simulink model "bsm2_ol_test"  (R2023b)
settings: Solver=ode15s  StartTime=0.0  StopTime=50  FixedStep=0.01  RelTol=1e-5  AbsTol=1e-8
values from neighbouring files (symbols this model uses):
  ACTIVATE = [ 0 ]    [init_bsm1.m]    (also in init_bsm2.m)
  carb1 = 0    [reginit_bsm1.m]    (also in reginit_bsm2.m = 2)
  carb2 = 0    [reginit_bsm1.m]    (also in reginit_bsm2.m)
  carb3 = 0    [reginit_bsm1.m]    (also in reginit_bsm2.m)
  carb4 = 0    [reginit_bsm1.m]    (also in reginit_bsm2.m)
  carb5 = 0    [reginit_bsm1.m]    (also in reginit_bsm2.m)
  KLa1 = 0    [reginit_bsm1.m]    (also in reginit_bsm2.m)
  KLa2 = 0    [reginit_bsm1.m]    (also in reginit_bsm2.m)
  KLa3 = 240    [reginit_bsm1.m]    (also in reginit_bsm2.m = 120)
  KLa4 = 240    [reginit_bsm1.m]    (also in reginit_bsm2.m = 120)
  KLa5 = 84    [reginit_bsm1.m]    (also in reginit_bsm2.m = 60)
  PAR_P = [ f_corr  f_X  t_m  f_PS ]    [primclarinit_bsm2.m]
  Qbypass = 60000    [reginit_bsm1.m]    (also in reginit_bsm2.m)
  QbypassAS = 0    [reginit_bsm1.m]    (also in reginit_bsm2.m)
  Qbypassplant = 1    [reginit_bsm1.m]    (also in reginit_bsm2.m)
  Qstorage = 0    [reginit_bsm1.m]    (also in reginit_bsm2.m)
  Qstorage2AS = 0    [reginit_bsm1.m]    (also in reginit_bsm2.m)
  Qthickener2AS = 0    [reginit_bsm1.m]    (also in reginit_bsm2.m)
  T = 0.0001    [hyddelayinit_bsm2.m]
  TEMPMODEL = [ 0 ]    [init_bsm1.m]    (also in init_bsm2.m)
  VOL_P = 900    [primclarinit_bsm2.m]
  XINIT_P = [ S_I_P  S_S_P  X_I_P  X_S_P  X_BH_P  X_BA_P  X_P_P  S_O_P  S_NO_P  S_NH_P  S_ND_P  X_ND_P  S_ALK_P TSS_P Q_P T_P S_D1_P S_D2_P S_D3_P X_D4_P X_D5_P ]    [primclarinit_bsm2.m]
  XINITDELAY = [ S_I_ASin  S_S_ASin  X_I_ASin  X_S_ASin  X_BH_ASin  X_BA_ASin  X_P_ASin  S_O_ASin  S_NO_ASin  S_NH_ASin  S_ND_ASin  X_ND_ASin  S_ALK_ASin TSS_ASin Q_ASin T_ASin S_D1_ASin S_D2_ASin S_D3_ASin X_D4_ASin X_D5_ASin ]    [hyddelayinit_bsm2.m]
  XINITDELAYPRIMARY = [ S_I_Pin  S_S_Pin  X_I_Pin  X_S_Pin  X_BH_Pin  X_BA_Pin  X_P_Pin  S_O_Pin  S_NO_Pin  S_NH_Pin  S_ND_Pin  X_ND_Pin  S_ALK_Pin TSS_Pin Q_Pin T_Pin S_D1_Pin S_D2_Pin S_D3_Pin X_D4_Pin X_D5_Pin ]    [hyddelayinit_bsm2.m]
  XVEKTOR_P = [0  0  1  1  1  1  1  0  0  0  0  1  0  0  0  0  0  0  0  1  1]    [primclarinit_bsm2.m]
undefined symbols (not defined in the file or in its folder): DIM, LAYER, MODELTYPE, PAR1, PAR2, PAR3, PAR4, PAR5, Qintr, Qr, Qw, SETTLERINIT, SETTLERPAR, SOSAT1, SOSAT2, SOSAT3, SOSAT4, SOSAT5, TIMEDELAY_S, VOL1, VOL2, VOL3, VOL4, VOL5, VOL_INIT_S, VOL_S, XINIT1, XINIT2, XINIT3, XINIT4, XINIT5, XINITSTORAGE
settings Model: Creator=ielulf  LastModifiedBy=miederer
settings SolverCC: AutoScaleAbsTol=off  AlgebraicLoopSolver=TrustRegion
settings DataIOCC: InitialState=xFinal  SaveFormat=Array  SignalLoggingSaveFormat=ModelDataLogs  SaveOutput=off  ReturnWorkspaceOutputs=off  TimeSaveName=t  SignalLoggingName=sigsOut  OutputOption=SpecifiedOutputTimes  OutputTimes=[0:(1/96):50]
settings OptimizationCC: BlockReduction=off  BooleanDataType=off  OptimizeBlockIOStorage=off  BufferReuse=off  GlobalBufferReuse=off  ExpressionFolding=off  LocalBlockOutputs=off  InitFltsAndDblsToZero=on  LifeSpan=inf  OptimizeDataStoreBuffers=off  BusAssignmentInplaceUpdate=off
settings DebuggingCC: SaveWithParameterizedLinksMsg=none  UnderspecifiedInitializationDetection=Classic  MergeDetectMultiDrivingBlocksExec=none  SignalResolutionControl=TryResolveAllWithWarning  InheritedTsInSrcMsg=none  MultiTaskDSMMsg=warning  MultiTaskCondExecSysMsg=none  FcnCallInpInsideContextMsg=warning  UnconnectedInputMsg=warning  UnconnectedLineMsg=warning  SFUnexpectedBacktrackingDiag=warning  SFNoUnconditionalDefaultTransitionDiag=warning  SFExecutionAtInitializationDiag=none  ArithmeticOperatorsInVariantConditions=warning
settings HardwareCC: ProdBitPerPointer=32  ProdBitPerSizeT=32  ProdBitPerPtrDiffT=32  ProdLargestAtomicFloat=None  ProdIntDivRoundTo=Undefined  ProdEndianess=Unspecified  ProdWordSize=32  ProdHWDeviceType=32-bit Generic  TargetUnknown=on
settings ModelReferenceCC: EnableRefExpFcnMdlSchedulingChecks=on  PropagateSignalLabelsOutOfModel=off
settings RTWCC: TemplateMakefile=grt_unix.tmf
settings CodeAppCC: StateflowObjectComments=on
settings GRTTargetCC: TargetFcnLib=ansi_tfl_tmw.mat  TargetLangStandard=C89/C90 (ANSI)  CombineOutputUpdateFcns=off  GRTInterface=on
settings ConfigComp: CovMetricSettings=dw  CovSaveCumulativeToWorkspaceVar=on  CovSaveSingleToWorkspaceVar=on

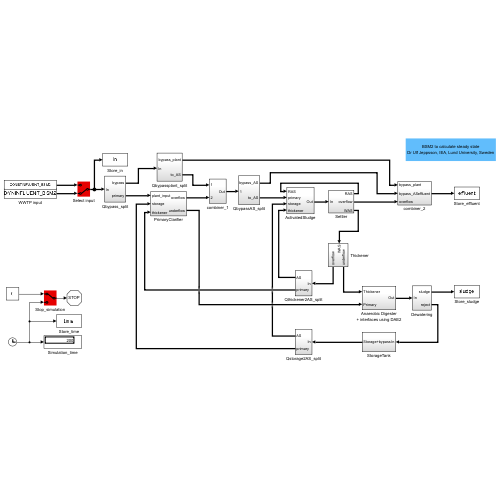
[thumbnail: Simulink's stored preview of the top-level diagram]
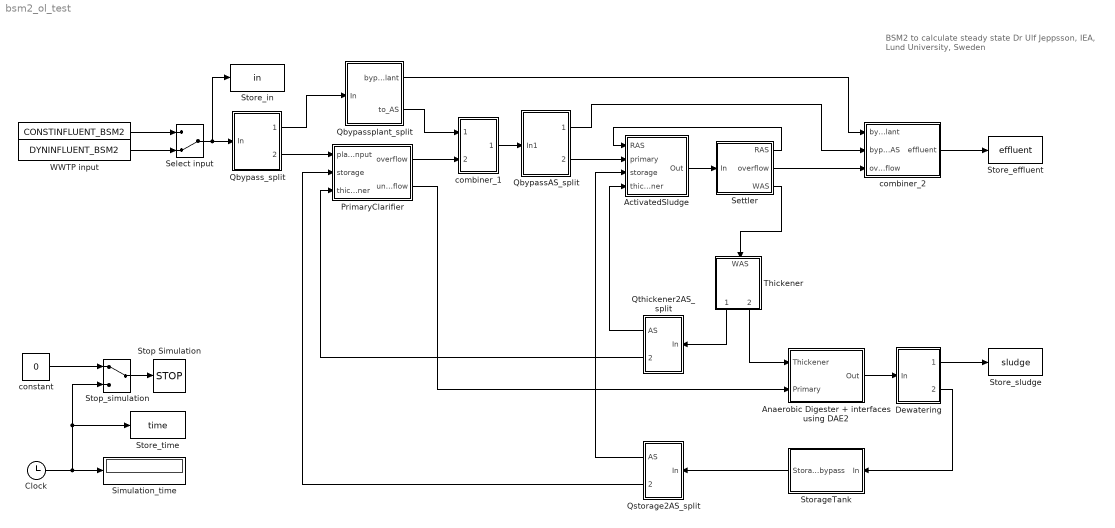
== system bsm2_ol_test ==
  note: BSM2 to calculate steady state
      |  Dr Ulf Jeppsson, IEA, Lund University, Sweden
  " " : FromWorkspace  VariableName=CONSTINFLUENT_BSM2  SampleTime=-1  ZeroCross=off  OutputAfterFinalValue=Holding final value
  " constant" : Constant  Value=0
  ActivatedSludge : Subsystem
  Anaerobic Digester + interfaces using DAE2 : Subsystem
  Clock : Clock
  Dewatering : Subsystem
  PrimaryClarifier : Subsystem
  QbypassAS_split : Subsystem
  Qbypass_split : Subsystem
  Qbypassplant_split : Subsystem
  Qstorage2AS_split : Subsystem
  Qthickener2AS_split : Subsystem
  Select input : ManualSwitch  CurrentSetting=0
  Settler : Subsystem
  Simulation_time : Display
  Stop Simulation : Stop
  Stop_simulation : ManualSwitch
  StorageTank : Subsystem
  Store_effluent : ToWorkspace  VariableName=effluent
  Store_in : ToWorkspace  VariableName=in
  Store_sludge : ToWorkspace  VariableName=sludge
  Store_time : ToWorkspace  VariableName=time
  Thickener : Subsystem
  WWTP input : FromWorkspace  VariableName=DYNINFLUENT_BSM2  SampleTime=-1  Interpolate=off  ZeroCross=off  OutputAfterFinalValue=Holding final value
  combiner_1 : Subsystem
  combiner_2 : Subsystem
  wires:
  ActivatedSludge/1(Out) -> Settler/1(In)
  Settler/1(RAS) -> ActivatedSludge/1(RAS)
  Settler/3(WAS) -> Thickener/1(WAS)
  Thickener/1(overflow) -> Qthickener2AS_split/1(In)
  Qthickener2AS_split/2(primary) -> PrimaryClarifier/3(thickener)
  Qthickener2AS_split/1(AS) -> ActivatedSludge/4(thickener)
  Qstorage2AS_split/1(AS) -> ActivatedSludge/3(storage)
  Qstorage2AS_split/2(primary) -> PrimaryClarifier/2(storage)
  Thickener/2(underflow) -> Anaerobic Digester + interfaces using DAE2/1(Thickener)
  Dewatering/2(reject) -> StorageTank/1(In)
  Dewatering/1(sludge) -> Store_sludge/1
  combiner_2/1(effluent) -> Store_effluent/1
  Settler/2(overflow) -> combiner_2/3(overflow)
  Qbypass_split/1(bypass) -> Qbypassplant_split/1(In)
  PrimaryClarifier/1(overflow) -> combiner_1/2(In2)
  combiner_1/1(Out) -> QbypassAS_split/1(In1)
  PrimaryClarifier/2(underflow) -> Anaerobic Digester + interfaces using DAE2/2(Primary)
  Anaerobic Digester + interfaces using DAE2/1(Out) -> Dewatering/1(In)
  Qbypass_split/2(primary) -> PrimaryClarifier/1(plant_input)
  Qbypassplant_split/2(to_AS) -> combiner_1/1(In1)
  Qbypassplant_split/1(bypass_plant) -> combiner_2/1(bypass_plant)
  QbypassAS_split/1(bypass_AS) -> combiner_2/2(bypass_AS)
  Clock/1 -> Simulation_time/1, Stop_simulation/2, Store_time/1
  Stop_simulation/1 -> Stop Simulation/1
  " constant"/1 -> Stop_simulation/1
  StorageTank/1(Storage+bypass) -> Qstorage2AS_split/1(In)
  QbypassAS_split/2(to_AS) -> ActivatedSludge/2(primary)
  Select input/1 -> Qbypass_split/1(In), Store_in/1
  " "/1 -> Select input/1
  WWTP input/1 -> Select input/2

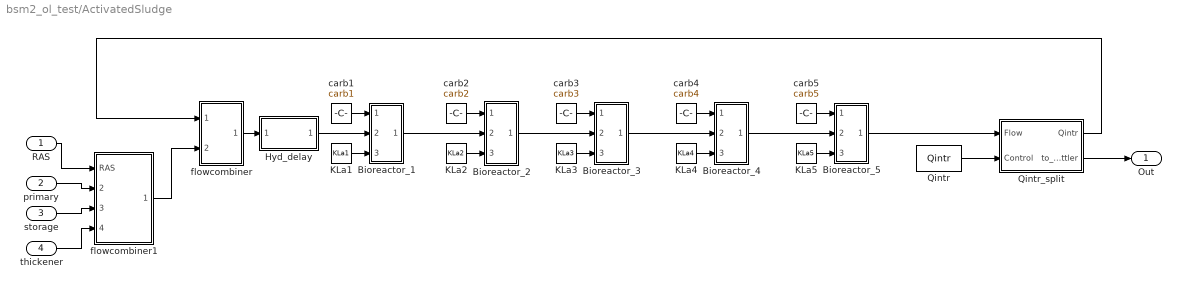
== system bsm2_ol_test/ActivatedSludge ==
  RAS : Inport
  primary : Inport  Port=2
  storage : Inport  Port=3
  thickener : Inport  Port=4
  Bioreactor_1 : Subsystem
  Bioreactor_2 : Subsystem
  Bioreactor_3 : Subsystem
  Bioreactor_4 : Subsystem
  Bioreactor_5 : Subsystem
  Hyd_delay : Subsystem
  KLa1 : Constant  Value=KLa1
  KLa2 : Constant  Value=KLa2
  KLa3 : Constant  Value=KLa3
  KLa4 : Constant  Value=KLa4
  KLa5 : Constant  Value=KLa5
  Qintr : Constant  Value=Qintr
  Qintr_split : Subsystem
  carb1 : Constant  Value=carb1
  carb2 : Constant  Value=carb2
  carb3 : Constant  Value=carb3
  carb4 : Constant  Value=carb4
  carb5 : Constant  Value=carb5
  flowcombiner : Subsystem
  flowcombiner1 : Subsystem
  Out : Outport
  wires:
  Qintr_split/1(Qintr) -> flowcombiner/1(Qintr)
  flowcombiner/1(Out) -> Hyd_delay/1(Input)
  Qintr_split/2(to_settler) -> Out/1
  RAS/1 -> flowcombiner1/1(RAS)
  storage/1 -> flowcombiner1/3(storage)
  thickener/1 -> flowcombiner1/4(thickener)
  primary/1 -> flowcombiner1/2(primary)
  Qintr/1 -> Qintr_split/2(Control)
  Bioreactor_5/1(out) -> Qintr_split/1(Flow)
  Hyd_delay/1(Output) -> Bioreactor_1/2(in)
  KLa1/1 -> Bioreactor_1/3(KLa)
  Bioreactor_1/1(out) -> Bioreactor_2/2(in)
  KLa2/1 -> Bioreactor_2/3(KLa)
  Bioreactor_2/1(out) -> Bioreactor_3/2(in)
  KLa3/1 -> Bioreactor_3/3(KLa)
  Bioreactor_3/1(out) -> Bioreactor_4/2(in)
  KLa4/1 -> Bioreactor_4/3(KLa)
  Bioreactor_4/1(out) -> Bioreactor_5/2(in)
  KLa5/1 -> Bioreactor_5/3(KLa)
  carb1/1 -> Bioreactor_1/1(carb)
  carb2/1 -> Bioreactor_2/1(carb)
  carb3/1 -> Bioreactor_3/1(carb)
  carb4/1 -> Bioreactor_4/1(carb)
  carb5/1 -> Bioreactor_5/1(carb)
  flowcombiner1/1(Out1) -> flowcombiner/2(Qin)

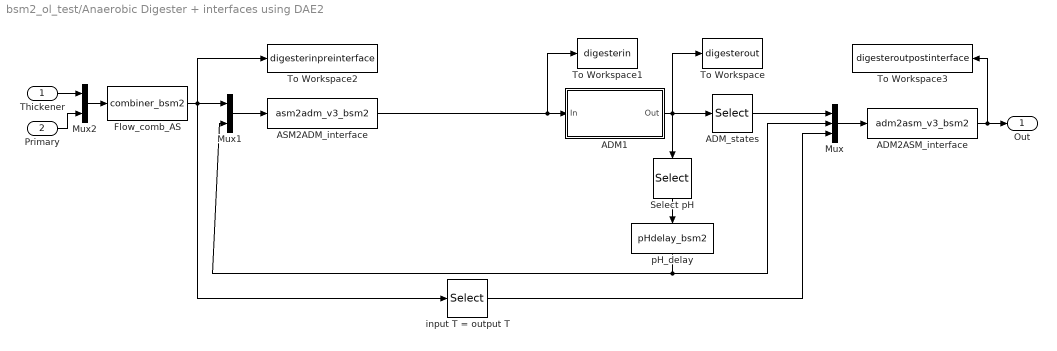
== system bsm2_ol_test/Anaerobic Digester + interfaces using DAE2 ==
  Thickener : Inport
  Primary : Inport  Port=2
  ADM1 : Subsystem
      mask Display: disp('adm1_DAE2_bsm2')
  ADM2ASM_interface : S-Function  FunctionName=adm2asm_v3_bsm2  Parameters=INTERFACEPAR  SFunctionDeploymentMode=off  EnableBusSupport=off
  ADM_states : Selector  InputPortWidth=51  IndexOptions=Index vector (dialog)  Indices=[1:33]  OutputSizes=1
  ASM2ADM_interface : S-Function  FunctionName=asm2adm_v3_bsm2  Parameters=INTERFACEPAR  SFunctionDeploymentMode=off  EnableBusSupport=off
  Flow_comb_AS : S-Function  FunctionName=combiner_bsm2  SFunctionDeploymentMode=off  EnableBusSupport=off
  Mux : Mux  Inputs=3
  Mux1 : Mux  Inputs=2
  Mux2 : Mux  Inputs=2
  Select pH : Selector  InputPortWidth=51  IndexOptions=Index vector (dialog)  Indices=[34]  OutputSizes=1
  To Workspace : ToWorkspace  VariableName=digesterout
  To Workspace1 : ToWorkspace  VariableName=digesterin
  To Workspace2 : ToWorkspace  VariableName=digesterinpreinterface
  To Workspace3 : ToWorkspace  VariableName=digesteroutpostinterface
  input T = output T : Selector  InputPortWidth=21  IndexOptions=Index vector (dialog)  Indices=[16]  OutputSizes=1
  pH_delay : S-Function  FunctionName=pHdelay_bsm2  Parameters=PHINIT, PHTIMECONST  SFunctionDeploymentMode=off  EnableBusSupport=off
  Out : Outport
  wires:
  ASM2ADM_interface/1 -> To Workspace1/1, ADM1/1(In)
  Primary/1 -> Mux2/2
  input T = output T/1 -> Mux/3
  Thickener/1 -> Mux2/1
  Mux2/1 -> Flow_comb_AS/1
  Flow_comb_AS/1 -> input T = output T/1, Mux1/1, To Workspace2/1
  pH_delay/1 -> Mux1/2, Mux/2
  ADM2ASM_interface/1 -> Out/1, To Workspace3/1
  Mux/1 -> ADM2ASM_interface/1
  ADM_states/1 -> Mux/1
  ADM1/1(Out) -> To Workspace/1, Select pH/1, ADM_states/1
  Mux1/1 -> ASM2ADM_interface/1
  Select pH/1 -> pH_delay/1

== system bsm2_ol_test/Dewatering ==
  In : Inport
  Dewatering : S-Function  FunctionName=dewatering_bsm2  Parameters=DEWATERINGPAR  SFunctionDeploymentMode=off  EnableBusSupport=off
  To Workspace1 : ToWorkspace  VariableName=dewateringout
  To Workspace11 : ToWorkspace  VariableName=dewateringin
  reject1 : Selector  InputPortWidth=42  IndexOptions=Index vector (dialog)  Indices=[22:42]  OutputSizes=1
  sludge1 : Selector  InputPortWidth=42  IndexOptions=Index vector (dialog)  Indices=[1:21]  OutputSizes=1
  sludge : Outport
  reject : Outport  Port=2
  wires:
  Dewatering/1 -> To Workspace1/1, reject1/1, sludge1/1
  In/1 -> Dewatering/1, To Workspace11/1
  sludge1/1 -> sludge/1
  reject1/1 -> reject/1

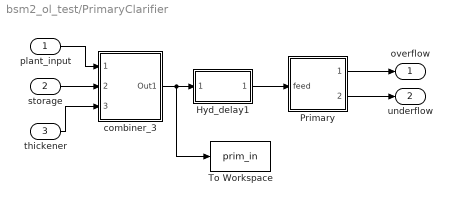
== system bsm2_ol_test/PrimaryClarifier ==
  plant_input : Inport
  storage : Inport  Port=2
  thickener : Inport  Port=3
  Hyd_delay1 : Subsystem
  Primary : Subsystem
  To Workspace : ToWorkspace  VariableName=prim_in
  combiner_3 : Subsystem
  overflow : Outport
  underflow : Outport  Port=2
  wires:
  Hyd_delay1/1(Output) -> Primary/1(feed)
  combiner_3/1(Out1) -> To Workspace/1, Hyd_delay1/1(Input)
  Primary/2(u_flow) -> underflow/1
  Primary/1(o_flow) -> overflow/1
  thickener/1 -> combiner_3/3(thickener)
  storage/1 -> combiner_3/2(storage)
  plant_input/1 -> combiner_3/1(sewerinput)

== system bsm2_ol_test/QbypassAS_split ==
  In1 : Inport
  FS_type_0 : Subsystem
  Store_qpassAS : ToWorkspace  VariableName=qpassAS
  To Workspace : ToWorkspace  VariableName=to_as
  flow_set : Constant  Value=QbypassAS
  bypass_AS : Outport
  to_AS : Outport  Port=2
  wires:
  flow_set/1 -> FS_type_0/2(Control)
  FS_type_0/1(bypass) -> bypass_AS/1, Store_qpassAS/1
  FS_type_0/2(main) -> to_AS/1, To Workspace/1
  In1/1 -> FS_type_0/1(Flow)

== system bsm2_ol_test/Qbypass_split ==
  In : Inport
  FS_type_2 : Subsystem
  Store_qpass : ToWorkspace  VariableName=qpass
  To Workspace : ToWorkspace  VariableName=to_primary
  flow1_set : Constant  Value=Qbypass
  bypass : Outport
  primary : Outport  Port=2
  wires:
  In/1 -> FS_type_2/1(Flow)
  FS_type_2/1(bypass) -> bypass/1, Store_qpass/1
  flow1_set/1 -> FS_type_2/2(Control)
  FS_type_2/2(main) -> To Workspace/1, primary/1

== system bsm2_ol_test/Qbypassplant_split ==
  In : Inport
  FS_type_0 : Subsystem
  Store_qpassplant : ToWorkspace  VariableName=qpassplant
  Store_qpassplant_to_as : ToWorkspace  VariableName=qpassplant_to_as
  flow1_set : Constant  Value=Qbypassplant
  bypass_plant : Outport
  to_AS : Outport  Port=2
  wires:
  In/1 -> FS_type_0/1(Flow)
  FS_type_0/1(bypass) -> bypass_plant/1, Store_qpassplant/1
  FS_type_0/2(main) -> Store_qpassplant_to_as/1, to_AS/1
  flow1_set/1 -> FS_type_0/2(Control)

== system bsm2_ol_test/Qstorage2AS_split ==
  In : Inport
  FS_type_0 : Subsystem
  Store_qstorage2AS : ToWorkspace  VariableName=qstorage2AS
  Store_qstorage2prim : ToWorkspace  VariableName=qstorage2prim
  flow1_set : Constant  Value=Qstorage2AS
  AS : Outport
  primary : Outport  Port=2
  wires:
  In/1 -> FS_type_0/1(Flow)
  FS_type_0/1(bypass) -> AS/1, Store_qstorage2AS/1
  FS_type_0/2(main) -> Store_qstorage2prim/1, primary/1
  flow1_set/1 -> FS_type_0/2(Control)

== system bsm2_ol_test/Qthickener2AS_split ==
  In : Inport
  FS_type_0 : Subsystem
  Store_qthick2AS : ToWorkspace  VariableName=qthick2AS
  Store_qthick2prim : ToWorkspace  VariableName=qthick2prim
  flow1_set : Constant  Value=Qthickener2AS
  AS : Outport
  primary : Outport  Port=2
  wires:
  In/1 -> FS_type_0/1(Flow)
  FS_type_0/1(bypass) -> AS/1, Store_qthick2AS/1
  flow1_set/1 -> FS_type_0/2(Control)
  FS_type_0/2(main) -> Store_qthick2prim/1, primary/1

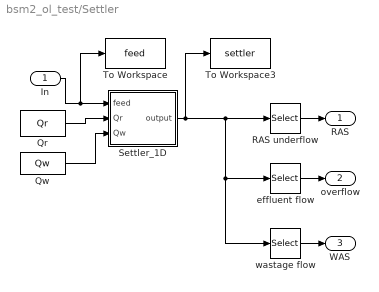
== system bsm2_ol_test/Settler ==
  In : Inport
  Qr : Constant  Value=Qr
  Qw : Constant  Value=Qw
  RAS underflow : Selector  InputPortWidth=166  IndexOptions=Index vector (dialog)  Indices=[1:21]  OutputSizes=1
  Settler_1D : Subsystem
  To Workspace : ToWorkspace  VariableName=feed
  To Workspace3 : ToWorkspace  VariableName=settler
  effluent flow : Selector  InputPortWidth=166  IndexOptions=Index vector (dialog)  Indices=[23:43]  OutputSizes=1
  wastage flow : Selector  InputPortWidth=166  IndexOptions=Index vector (dialog)  Indices=[1:14,22,16:21]  OutputSizes=1
  RAS : Outport
  overflow : Outport  Port=2
  WAS : Outport  Port=3
  wires:
  In/1 -> To Workspace/1, Settler_1D/1(feed)
  Settler_1D/1(output) -> RAS underflow/1, effluent flow/1, wastage flow/1, To Workspace3/1
  wastage flow/1 -> WAS/1
  effluent flow/1 -> overflow/1
  RAS underflow/1 -> RAS/1
  Qr/1 -> Settler_1D/2(Qr)
  Qw/1 -> Settler_1D/3(Qw)

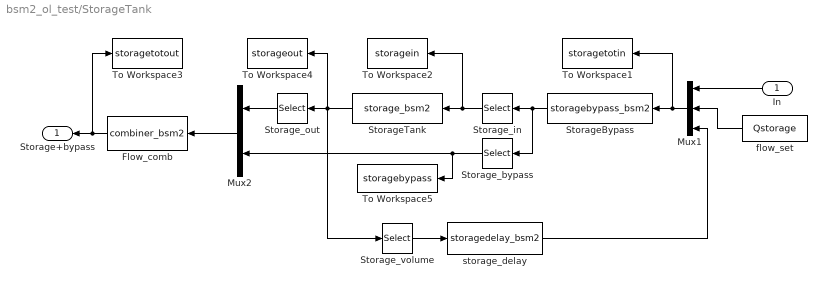
== system bsm2_ol_test/StorageTank ==
  In : Inport
  Flow_comb : S-Function  FunctionName=combiner_bsm2  SFunctionDeploymentMode=off  EnableBusSupport=off
  Mux1 : Mux  Inputs=3
  Mux2 : Mux  Inputs=2
  StorageBypass : S-Function  FunctionName=storagebypass_bsm2  Parameters=VOL_S  SFunctionDeploymentMode=off  EnableBusSupport=off
  StorageTank : S-Function  FunctionName=storage_bsm2  Parameters=XINITSTORAGE,VOL_S,TEMPMODEL,ACTIVATE  SFunctionDeploymentMode=off  EnableBusSupport=off
  Storage_bypass : Selector  InputPortWidth=43  IndexOptions=Index vector (dialog)  Indices=[23:43]  OutputSizes=1
  Storage_in : Selector  InputPortWidth=43  IndexOptions=Index vector (dialog)  Indices=[1:22]  OutputSizes=1
  Storage_out : Selector  InputPortWidth=22  IndexOptions=Index vector (dialog)  Indices=[1:21]  OutputSizes=1
  Storage_volume : Selector  InputPortWidth=22  IndexOptions=Index vector (dialog)  Indices=[22]  OutputSizes=1
  To Workspace1 : ToWorkspace  VariableName=storagetotin
  To Workspace2 : ToWorkspace  VariableName=storagein
  To Workspace3 : ToWorkspace  VariableName=storagetotout
  To Workspace4 : ToWorkspace  VariableName=storageout
  To Workspace5 : ToWorkspace  VariableName=storagebypass
  flow_set : Constant  Value=Qstorage
  storage_delay : S-Function  FunctionName=storagedelay_bsm2  Parameters=VOL_INIT_S,TIMEDELAY_S  SFunctionDeploymentMode=off  EnableBusSupport=off
  Storage+bypass : Outport
  wires:
  Flow_comb/1 -> Storage+bypass/1, To Workspace3/1
  Storage_volume/1 -> storage_delay/1
  In/1 -> Mux1/1
  Storage_out/1 -> Mux2/1
  StorageTank/1 -> Storage_volume/1, To Workspace4/1, Storage_out/1
  Storage_bypass/1 -> To Workspace5/1, Mux2/2
  Storage_in/1 -> To Workspace2/1, StorageTank/1
  Mux2/1 -> Flow_comb/1
  StorageBypass/1 -> Storage_bypass/1, Storage_in/1
  flow_set/1 -> Mux1/2
  Mux1/1 -> To Workspace1/1, StorageBypass/1
  storage_delay/1 -> Mux1/3

== system bsm2_ol_test/Thickener ==
  WAS : Inport
  Thickener : Subsystem
  overflow : Outport
  underflow : Outport  Port=2
  wires:
  WAS/1 -> Thickener/1(feed)
  Thickener/1(o_flow) -> overflow/1
  Thickener/2(u_flow) -> underflow/1

== system bsm2_ol_test/combiner_1 ==
  In1 : Inport
  In2 : Inport  Port=2
  Flow_comb2 : S-Function  FunctionName=combiner_bsm2  SFunctionDeploymentMode=off  EnableBusSupport=off
  bypass1 and primary : Mux  Inputs=2
  Out : Outport
  wires:
  bypass1 and primary/1 -> Flow_comb2/1
  In1/1 -> bypass1 and primary/1
  Flow_comb2/1 -> Out/1
  In2/1 -> bypass1 and primary/2

== system bsm2_ol_test/combiner_2 ==
  bypass_plant : Inport
  bypass_AS : Inport  Port=2
  overflow : Inport  Port=3
  3_streams : Mux  Inputs=3
  Flow_comb3 : S-Function  FunctionName=combiner3_bsm2  SFunctionDeploymentMode=off  EnableBusSupport=off
  effluent : Outport
  wires:
  3_streams/1 -> Flow_comb3/1
  Flow_comb3/1 -> effluent/1
  overflow/1 -> 3_streams/1
  bypass_plant/1 -> 3_streams/2
  bypass_AS/1 -> 3_streams/3

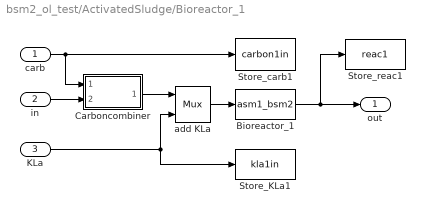
== system bsm2_ol_test/ActivatedSludge/Bioreactor_1 ==
  carb : Inport
  in : Inport  Port=2
  KLa : Inport  Port=3
  Bioreactor_1 : S-Function  FunctionName=asm1_bsm2  Parameters=XINIT1,PAR1,VOL1,SOSAT1,TEMPMODEL,ACTIVATE  SFunctionDeploymentMode=off  EnableBusSupport=off
  Carboncombiner : Subsystem
  Store_KLa1 : ToWorkspace  VariableName=kla1in  SampleTime=-1
  Store_carb1 : ToWorkspace  VariableName=carbon1in  SampleTime=-1
  Store_reac1 : ToWorkspace  VariableName=reac1  SampleTime=-1
  add KLa : Mux  Inputs=2
  out : Outport
  wires:
  KLa/1 -> Store_KLa1/1, add KLa/2
  in/1 -> Carboncombiner/2(Input)
  carb/1 -> Carboncombiner/1(C_flow), Store_carb1/1
  Carboncombiner/1(Output) -> add KLa/1
  Bioreactor_1/1 -> Store_reac1/1, out/1
  add KLa/1 -> Bioreactor_1/1

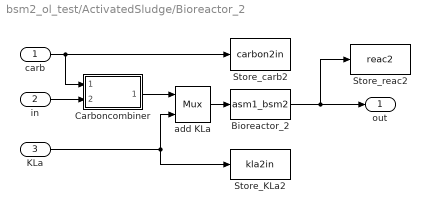
== system bsm2_ol_test/ActivatedSludge/Bioreactor_2 ==
  carb : Inport
  in : Inport  Port=2
  KLa : Inport  Port=3
  Bioreactor_2 : S-Function  FunctionName=asm1_bsm2  Parameters=XINIT2,PAR2,VOL2,SOSAT2,TEMPMODEL,ACTIVATE  SFunctionDeploymentMode=off  EnableBusSupport=off
  Carboncombiner : Subsystem
  Store_KLa2 : ToWorkspace  VariableName=kla2in  SampleTime=-1
  Store_carb2 : ToWorkspace  VariableName=carbon2in  SampleTime=-1
  Store_reac2 : ToWorkspace  VariableName=reac2  SampleTime=-1
  add KLa : Mux  Inputs=2
  out : Outport
  wires:
  KLa/1 -> Store_KLa2/1, add KLa/2
  in/1 -> Carboncombiner/2(Input)
  carb/1 -> Store_carb2/1, Carboncombiner/1(C_flow)
  Carboncombiner/1(Output) -> add KLa/1
  add KLa/1 -> Bioreactor_2/1
  Bioreactor_2/1 -> Store_reac2/1, out/1

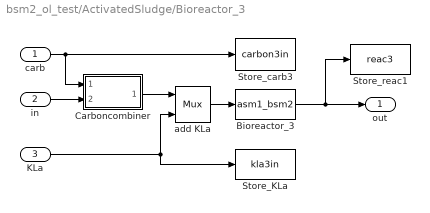
== system bsm2_ol_test/ActivatedSludge/Bioreactor_3 ==
  carb : Inport
  in : Inport  Port=2
  KLa : Inport  Port=3
  Bioreactor_3 : S-Function  FunctionName=asm1_bsm2  Parameters=XINIT3,PAR3,VOL3,SOSAT3,TEMPMODEL,ACTIVATE  SFunctionDeploymentMode=off  EnableBusSupport=off
  Carboncombiner : Subsystem
  Store_KLa : ToWorkspace  VariableName=kla3in  SampleTime=-1
  Store_carb3 : ToWorkspace  VariableName=carbon3in  SampleTime=-1
  Store_reac1 : ToWorkspace  VariableName=reac3  SampleTime=-1
  add KLa : Mux  Inputs=2
  out : Outport
  wires:
  KLa/1 -> Store_KLa/1, add KLa/2
  in/1 -> Carboncombiner/2(Input)
  carb/1 -> Store_carb3/1, Carboncombiner/1(C_flow)
  Carboncombiner/1(Output) -> add KLa/1
  add KLa/1 -> Bioreactor_3/1
  Bioreactor_3/1 -> Store_reac1/1, out/1

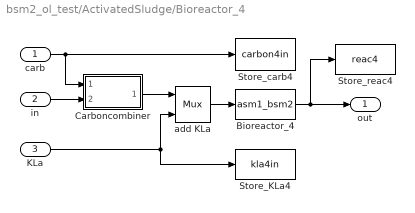
== system bsm2_ol_test/ActivatedSludge/Bioreactor_4 ==
  carb : Inport
  in : Inport  Port=2
  KLa : Inport  Port=3
  Bioreactor_4 : S-Function  FunctionName=asm1_bsm2  Parameters=XINIT4,PAR4,VOL4,SOSAT4,TEMPMODEL,ACTIVATE  SFunctionDeploymentMode=off  EnableBusSupport=off
  Carboncombiner : Subsystem
  Store_KLa4 : ToWorkspace  VariableName=kla4in  SampleTime=-1
  Store_carb4 : ToWorkspace  VariableName=carbon4in  SampleTime=-1
  Store_reac4 : ToWorkspace  VariableName=reac4  SampleTime=-1
  add KLa : Mux  Inputs=2
  out : Outport
  wires:
  KLa/1 -> Store_KLa4/1, add KLa/2
  in/1 -> Carboncombiner/2(Input)
  carb/1 -> Store_carb4/1, Carboncombiner/1(C_flow)
  Carboncombiner/1(Output) -> add KLa/1
  add KLa/1 -> Bioreactor_4/1
  Bioreactor_4/1 -> Store_reac4/1, out/1

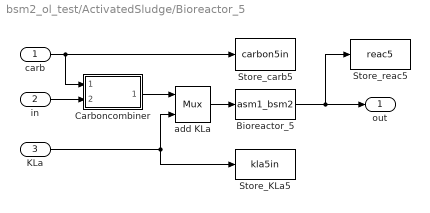
== system bsm2_ol_test/ActivatedSludge/Bioreactor_5 ==
  carb : Inport
  in : Inport  Port=2
  KLa : Inport  Port=3
  Bioreactor_5 : S-Function  FunctionName=asm1_bsm2  Parameters=XINIT5,PAR5,VOL5,SOSAT5,TEMPMODEL,ACTIVATE  SFunctionDeploymentMode=off  EnableBusSupport=off
  Carboncombiner : Subsystem
  Store_KLa5 : ToWorkspace  VariableName=kla5in  SampleTime=-1
  Store_carb5 : ToWorkspace  VariableName=carbon5in  SampleTime=-1
  Store_reac5 : ToWorkspace  VariableName=reac5  SampleTime=-1
  add KLa : Mux  Inputs=2
  out : Outport
  wires:
  KLa/1 -> Store_KLa5/1, add KLa/2
  in/1 -> Carboncombiner/2(Input)
  carb/1 -> Store_carb5/1, Carboncombiner/1(C_flow)
  Carboncombiner/1(Output) -> add KLa/1
  add KLa/1 -> Bioreactor_5/1
  Bioreactor_5/1 -> Store_reac5/1, out/1

== system bsm2_ol_test/ActivatedSludge/Hyd_delay ==
  Input : Inport
  Demux : Demux  Outputs=[14,1,1,5]
      settings: DisplayOption=none
  Hyd_delay : S-Function  FunctionName=hyddelayv3_bsm2  Parameters=XINITDELAY,PAR1,T  SFunctionDeploymentMode=off  EnableBusSupport=off
  Massinput_g/d : ToWorkspace  VariableName=ASinput  SampleTime=-1
  Mux : Mux
  Product : Product  SaturateOnIntegerOverflow=on  OutDataTypeStr=Inherit: Same as first input
  Product1 : Product  SaturateOnIntegerOverflow=on  OutDataTypeStr=Inherit: Same as first input
  Output : Outport
  wires:
  Mux/1 -> Massinput_g/d/1
  Product/1 -> Mux/1
  Demux/1 -> Product/1
  Hyd_delay/1 -> Output/1, Demux/1
  Input/1 -> Hyd_delay/1
  Demux/2 -> Product/2, Mux/2, Product1/1
  Demux/3 -> Mux/3
  Product1/1 -> Mux/4
  Demux/4 -> Product1/2

== system bsm2_ol_test/ActivatedSludge/Qintr_split ==
  Flow : Inport
  Control : Inport  Port=2
  Flow_splitter_type1 : S-Function  FunctionName=flowsplitter_bsm2  Parameters=Qintrtype  SFunctionDeploymentMode=off  EnableBusSupport=off
  Mux1 : Mux  Inputs=2
  Selector : Selector  InputPortWidth=42  IndexOptions=Index vector (dialog)  Indices=[1:21]  OutputSizes=1
  Selector1 : Selector  InputPortWidth=42  IndexOptions=Index vector (dialog)  Indices=[22:42]  OutputSizes=1
  Qintr : Outport
  to_settler : Outport  Port=2
  wires:
  Selector1/1 -> to_settler/1
  Control/1 -> Mux1/2
  Flow/1 -> Mux1/1
  Selector/1 -> Qintr/1
  Mux1/1 -> Flow_splitter_type1/1
  Flow_splitter_type1/1 -> Selector1/1, Selector/1

== system bsm2_ol_test/ActivatedSludge/flowcombiner ==
  Qintr : Inport
  Qin : Inport  Port=2
  Flow_comb2 : S-Function  FunctionName=combiner_bsm2  SFunctionDeploymentMode=off  EnableBusSupport=off
  Qin and Qintr : Mux  Inputs=2
  Store_rec : ToWorkspace  VariableName=rec
  Out : Outport
  wires:
  Qin and Qintr/1 -> Flow_comb2/1
  Qintr/1 -> Qin and Qintr/1, Store_rec/1
  Flow_comb2/1 -> Out/1
  Qin/1 -> Qin and Qintr/2

== system bsm2_ol_test/ActivatedSludge/flowcombiner1 ==
  RAS : Inport
  primary : Inport  Port=2
  storage : Inport  Port=3
  thickener : Inport  Port=4
  4_streams : Mux
  Flow_comb4 : S-Function  FunctionName=combiner4_bsm2  SFunctionDeploymentMode=off  EnableBusSupport=off
  Out1 : Outport
  wires:
  4_streams/1 -> Flow_comb4/1
  RAS/1 -> 4_streams/1
  Flow_comb4/1 -> Out1/1
  primary/1 -> 4_streams/2
  storage/1 -> 4_streams/3
  thickener/1 -> 4_streams/4

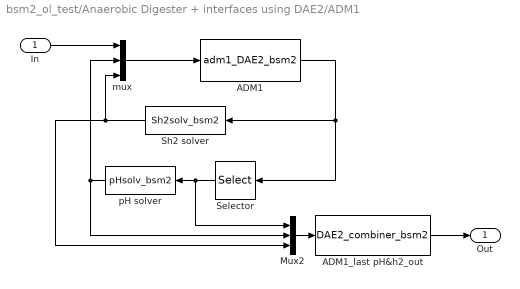
== system bsm2_ol_test/Anaerobic Digester + interfaces using DAE2/ADM1 ==
  In : Inport
  ADM1 : S-Function  FunctionName=adm1_DAE2_bsm2  Parameters=DIGESTERINIT, DIGESTERPAR, DIM_D  SFunctionDeploymentMode=off  EnableBusSupport=off
  ADM1_last pH&h2_out : S-Function  FunctionName=DAE2_combiner_bsm2  SFunctionDeploymentMode=off  EnableBusSupport=off
  Mux2 : Mux  Inputs=3
  Selector : Selector  InputPortWidth=52  IndexOptions=Index vector (dialog)  Indices=[1:51]  OutputSizes=1
  Sh2 solver : S-Function  FunctionName=Sh2solv_bsm2  Parameters=SH2SOLVINIT, DIGESTERPAR, DIM_D  SFunctionDeploymentMode=off  EnableBusSupport=off
  mux : Mux  Inputs=3
  pH solver : S-Function  FunctionName=pHsolv_bsm2  Parameters=PHSOLVINIT, DIGESTERPAR  SFunctionDeploymentMode=off  EnableBusSupport=off
  Out : Outport
  wires:
  ADM1_last pH&h2_out/1 -> Out/1
  Mux2/1 -> ADM1_last pH&h2_out/1
  pH solver/1 -> Mux2/2, mux/2
  ADM1/1 -> Sh2 solver/1, Selector/1
  In/1 -> mux/1
  mux/1 -> ADM1/1
  Sh2 solver/1 -> Mux2/3, mux/3
  Selector/1 -> Mux2/1, pH solver/1

== system bsm2_ol_test/PrimaryClarifier/Hyd_delay1 ==
  Input : Inport
  Demux : Demux  Outputs=[14,1,1,5]
      settings: DisplayOption=none
  Hyd_delay : S-Function  FunctionName=hyddelayv3_bsm2  Parameters=XINITDELAYPRIMARY,PAR1,T  SFunctionDeploymentMode=off  EnableBusSupport=off
  Massinput_g/d : ToWorkspace  VariableName=primaryinput  SampleTime=-1
  Mux : Mux
  Product : Product  SaturateOnIntegerOverflow=on  OutDataTypeStr=Inherit: Same as first input
  Product1 : Product  SaturateOnIntegerOverflow=on  OutDataTypeStr=Inherit: Same as first input
  Output : Outport
  wires:
  Demux/4 -> Product1/2
  Product1/1 -> Mux/4
  Demux/3 -> Mux/3
  Demux/2 -> Product1/1, Mux/2, Product/2
  Input/1 -> Hyd_delay/1
  Hyd_delay/1 -> Demux/1, Output/1
  Demux/1 -> Product/1
  Product/1 -> Mux/1
  Mux/1 -> Massinput_g/d/1

== system bsm2_ol_test/PrimaryClarifier/Primary ==
  feed : Inport
  Primary Clarifier : S-Function  FunctionName=primclar_bsm2  Parameters=XINIT_P,XVEKTOR_P,PAR_P,VOL_P,PAR1,TEMPMODEL  SFunctionDeploymentMode=off  EnableBusSupport=off
  Store_primaryin : ToWorkspace  VariableName=primaryin
  Store_primaryout : ToWorkspace  VariableName=primaryout
  overflow : Selector  InputPortWidth=63  IndexOptions=Index vector (dialog)  Indices=[1:21]  OutputSizes=1
  underflow : Selector  InputPortWidth=63  IndexOptions=Index vector (dialog)  Indices=[22:42]  OutputSizes=1
  o_flow : Outport
  u_flow : Outport  Port=2
  wires:
  Primary Clarifier/1 -> Store_primaryout/1, underflow/1, overflow/1
  feed/1 -> Primary Clarifier/1, Store_primaryin/1
  underflow/1 -> u_flow/1
  overflow/1 -> o_flow/1

== system bsm2_ol_test/PrimaryClarifier/combiner_3 ==
  sewerinput : Inport
  storage : Inport  Port=2
  thickener : Inport  Port=3
  3_streams : Mux  Inputs=3
  Flow_comb3 : S-Function  FunctionName=combiner3_bsm2  SFunctionDeploymentMode=off  EnableBusSupport=off
  Out1 : Outport
  wires:
  3_streams/1 -> Flow_comb3/1
  sewerinput/1 -> 3_streams/1
  Flow_comb3/1 -> Out1/1
  storage/1 -> 3_streams/2
  thickener/1 -> 3_streams/3

== system bsm2_ol_test/QbypassAS_split/FS_type_0 ==
  Flow : Inport
  Control : Inport  Port=2
  Flow_splitter_type0 : S-Function  FunctionName=flowsplitter_bsm2  Parameters=QbypassAStype  SFunctionDeploymentMode=off  EnableBusSupport=off
  Mux1 : Mux  Inputs=2
  Selector : Selector  InputPortWidth=42  IndexOptions=Index vector (dialog)  Indices=[1:21]  OutputSizes=1
  Selector1 : Selector  InputPortWidth=42  IndexOptions=Index vector (dialog)  Indices=[22:42]  OutputSizes=1
  bypass : Outport
  main : Outport  Port=2
  wires:
  Selector1/1 -> main/1
  Control/1 -> Mux1/2
  Flow/1 -> Mux1/1
  Selector/1 -> bypass/1
  Mux1/1 -> Flow_splitter_type0/1
  Flow_splitter_type0/1 -> Selector1/1, Selector/1

== system bsm2_ol_test/Qbypass_split/FS_type_2 ==
  Flow : Inport
  Control : Inport  Port=2
  Flow_splitter_type2 : S-Function  FunctionName=flowsplitter_bsm2  Parameters=Qbypasstype  SFunctionDeploymentMode=off  EnableBusSupport=off
  Mux1 : Mux  Inputs=2
  Selector : Selector  InputPortWidth=42  IndexOptions=Index vector (dialog)  Indices=[1:21]  OutputSizes=1
  Selector1 : Selector  InputPortWidth=42  IndexOptions=Index vector (dialog)  Indices=[22:42]  OutputSizes=1
  bypass : Outport
  main : Outport  Port=2
  wires:
  Selector1/1 -> main/1
  Control/1 -> Mux1/2
  Flow/1 -> Mux1/1
  Selector/1 -> bypass/1
  Mux1/1 -> Flow_splitter_type2/1
  Flow_splitter_type2/1 -> Selector1/1, Selector/1

== system bsm2_ol_test/Qbypassplant_split/FS_type_0 ==
  Flow : Inport
  Control : Inport  Port=2
  Flow_splitter_type0 : S-Function  FunctionName=flowsplitter_bsm2  Parameters=Qbypassplanttype  SFunctionDeploymentMode=off  EnableBusSupport=off
  Mux1 : Mux  Inputs=2
  Selector : Selector  InputPortWidth=42  IndexOptions=Index vector (dialog)  Indices=[1:21]  OutputSizes=1
  Selector1 : Selector  InputPortWidth=42  IndexOptions=Index vector (dialog)  Indices=[22:42]  OutputSizes=1
  bypass : Outport
  main : Outport  Port=2
  wires:
  Selector1/1 -> main/1
  Control/1 -> Mux1/2
  Flow/1 -> Mux1/1
  Selector/1 -> bypass/1
  Mux1/1 -> Flow_splitter_type0/1
  Flow_splitter_type0/1 -> Selector1/1, Selector/1

== system bsm2_ol_test/Qstorage2AS_split/FS_type_0 ==
  Flow : Inport
  Control : Inport  Port=2
  Flow_splitter_type0 : S-Function  FunctionName=flowsplitter_bsm2  Parameters=Qstorage2AStype  SFunctionDeploymentMode=off  EnableBusSupport=off
  Mux1 : Mux  Inputs=2
  Selector : Selector  InputPortWidth=42  IndexOptions=Index vector (dialog)  Indices=[1:21]  OutputSizes=1
  Selector1 : Selector  InputPortWidth=42  IndexOptions=Index vector (dialog)  Indices=[22:42]  OutputSizes=1
  bypass : Outport
  main : Outport  Port=2
  wires:
  Selector1/1 -> main/1
  Control/1 -> Mux1/2
  Flow/1 -> Mux1/1
  Selector/1 -> bypass/1
  Mux1/1 -> Flow_splitter_type0/1
  Flow_splitter_type0/1 -> Selector1/1, Selector/1

== system bsm2_ol_test/Qthickener2AS_split/FS_type_0 ==
  Flow : Inport
  Control : Inport  Port=2
  Flow_splitter_type0 : S-Function  FunctionName=flowsplitter_bsm2  Parameters=Qthickener2AStype  SFunctionDeploymentMode=off  EnableBusSupport=off
  Mux1 : Mux  Inputs=2
  Selector : Selector  InputPortWidth=42  IndexOptions=Index vector (dialog)  Indices=[1:21]  OutputSizes=1
  Selector1 : Selector  InputPortWidth=42  IndexOptions=Index vector (dialog)  Indices=[22:42]  OutputSizes=1
  bypass : Outport
  main : Outport  Port=2
  wires:
  Selector1/1 -> main/1
  Control/1 -> Mux1/2
  Flow/1 -> Mux1/1
  Selector/1 -> bypass/1
  Mux1/1 -> Flow_splitter_type0/1
  Flow_splitter_type0/1 -> Selector1/1, Selector/1

== system bsm2_ol_test/Settler/Settler_1D ==
  feed : Inport
  Qr : Inport  Port=2
  Qw : Inport  Port=3
  Settler_1D : S-Function  FunctionName=settler1dv5_bsm2  Parameters=SETTLERINIT,SETTLERPAR,DIM,LAYER,MODELTYPE,TEMPMODEL,ACTIVATE  SFunctionDeploymentMode=off  EnableBusSupport=off
  add Qr and Qw : Mux  Inputs=3
  output : Outport
  wires:
  Settler_1D/1 -> output/1
  feed/1 -> add Qr and Qw/1
  Qw/1 -> add Qr and Qw/3
  Qr/1 -> add Qr and Qw/2
  add Qr and Qw/1 -> Settler_1D/1

== system bsm2_ol_test/Thickener/Thickener ==
  feed : Inport
  Thickener : S-Function  FunctionName=thickener_bsm2  Parameters=THICKENERPAR  SFunctionDeploymentMode=off  EnableBusSupport=off
  To Workspace1 : ToWorkspace  VariableName=thickenerin
  To Workspace11 : ToWorkspace  VariableName=thickenerout
  overflow : Selector  InputPortWidth=42  IndexOptions=Index vector (dialog)  Indices=[22:42]  OutputSizes=1
  underflow : Selector  InputPortWidth=42  IndexOptions=Index vector (dialog)  Indices=[1:21]  OutputSizes=1
  o_flow : Outport
  u_flow : Outport  Port=2
  wires:
  feed/1 -> To Workspace1/1, Thickener/1
  Thickener/1 -> overflow/1, underflow/1, To Workspace11/1
  overflow/1 -> o_flow/1
  underflow/1 -> u_flow/1

== system bsm2_ol_test/ActivatedSludge/Bioreactor_1/Carboncombiner ==
  C_flow : Inport
  Input : Inport  Port=2
  Carboncombiner : S-Function  FunctionName=carboncombiner_bsm2  Parameters=CARBONSOURCECONC  SFunctionDeploymentMode=off  EnableBusSupport=off
  Mux : Mux  Inputs=2
  Output : Outport
  wires:
  Input/1 -> Mux/2
  Carboncombiner/1 -> Output/1
  Mux/1 -> Carboncombiner/1
  C_flow/1 -> Mux/1

== system bsm2_ol_test/ActivatedSludge/Bioreactor_2/Carboncombiner ==
  C_flow : Inport
  Input : Inport  Port=2
  Carboncombiner : S-Function  FunctionName=carboncombiner_bsm2  Parameters=CARBONSOURCECONC  SFunctionDeploymentMode=off  EnableBusSupport=off
  Mux : Mux  Inputs=2
  Output : Outport
  wires:
  C_flow/1 -> Mux/1
  Mux/1 -> Carboncombiner/1
  Carboncombiner/1 -> Output/1
  Input/1 -> Mux/2

== system bsm2_ol_test/ActivatedSludge/Bioreactor_3/Carboncombiner ==
  C_flow : Inport
  Input : Inport  Port=2
  Carboncombiner : S-Function  FunctionName=carboncombiner_bsm2  Parameters=CARBONSOURCECONC  SFunctionDeploymentMode=off  EnableBusSupport=off
  Mux : Mux  Inputs=2
  Output : Outport
  wires:
  C_flow/1 -> Mux/1
  Mux/1 -> Carboncombiner/1
  Carboncombiner/1 -> Output/1
  Input/1 -> Mux/2

== system bsm2_ol_test/ActivatedSludge/Bioreactor_4/Carboncombiner ==
  C_flow : Inport
  Input : Inport  Port=2
  Carboncombiner : S-Function  FunctionName=carboncombiner_bsm2  Parameters=CARBONSOURCECONC  SFunctionDeploymentMode=off  EnableBusSupport=off
  Mux : Mux  Inputs=2
  Output : Outport
  wires:
  C_flow/1 -> Mux/1
  Mux/1 -> Carboncombiner/1
  Carboncombiner/1 -> Output/1
  Input/1 -> Mux/2

== system bsm2_ol_test/ActivatedSludge/Bioreactor_5/Carboncombiner ==
  C_flow : Inport
  Input : Inport  Port=2
  Carboncombiner : S-Function  FunctionName=carboncombiner_bsm2  Parameters=CARBONSOURCECONC  SFunctionDeploymentMode=off  EnableBusSupport=off
  Mux : Mux  Inputs=2
  Output : Outport
  wires:
  C_flow/1 -> Mux/1
  Mux/1 -> Carboncombiner/1
  Carboncombiner/1 -> Output/1
  Input/1 -> Mux/2
